simulink model "Copy_of_MPC_control"  (R2018a)
settings: Solver=FixedStepAuto  StartTime=0  StopTime=Tend  FixedStep=0.001  RelTol=5e-3
model workspace (MAT data in the model file):
  A_mu = 10
  B_reff = 8.386
  Cz = 7766.25
  DCT_Param : struct (value not decoded)
  D_reff = 0.25826
  Downshift_Speeds = [9.5625 12.9375 16.3125 19.6875 23.0625 26.4375 29.8125 33.1875 36.5625 39.9375 43.3125 46.6875 ... (28 elements, 4x7)]
  Pedal_Positions = [0.1 0.4 0.5 0.9]
  SUS : struct (value not decoded)
  Upshift_Speeds = [12.9375 16.3125 19.6875 33 26.4375 29.8125 33.1875 52.5 39.9375 43.3125 46.6875 77.25 ... (28 elements, 4x7)]
  VEH : struct (value not decoded)
  V_o = 16.7
  V_xlow = 1
  WH : struct (value not decoded)
  a = 1.4
  alpha_max = 1.5
  alpha_min = -1.5
  b = 1.8
  c_zo = 209651
  epsilon = 0.1
  h = 0.134
  path : struct (value not decoded)
  pio = 220000
  q_Fcx = 0
  q_Fz2 = 15.4
  q_Fzy = 0
  q_reo = 0.9974
  q_sx1 = -0.007764
  q_sx10 = 0.2824
  q_sx11 = 5.349
  q_sx12 = 0
  q_sx13 = 0
  q_sx14 = 0
  q_sx2 = 1.1915
  q_sx3 = 0.013948
  q_sx4 = 4.912
  q_sx5 = 1.02
  q_sx6 = 22.83
  q_sx7 = 0.7104
  q_sx8 = -0.023393
  q_sx9 = 0.6581
  q_sy1 = 0.00702
  q_sy2 = 0
  q_sy3 = 0.001515
  q_sy4 = 8.514e-05
  q_sy5 = 0
  q_sy6 = 0
  q_sy7 = 0.9008
  q_sy8 = -0.4089
  q_v1 = 0.0007742
  q_v2 = 0.04667
  r_Bx1 = 12.531
  r_Bx2 = 9.532
  r_Bx3 = 0
  r_By1 = 10.615
  r_By2 = 7.705
  r_By3 = 3.433e-06
  r_By4 = 0
  r_Cx1 = 1.019
  r_Cy1 = 1.0585
  r_Ex1 = -0.4487
  r_Ex2 = -0.4726
  r_Ey1 = 0.3132
  r_Ey2 = 7.63e-06
  r_Hx1 = 0.0002374
  r_Hy1 = 0.011646
  r_Hy2 = 7.63e-06
  r_Vy1 = 0.05654
  r_Vy2 = 7.63e-06
  r_Vy3 = 0
  r_Vy4 = 99.9
  r_Vy5 = 2
  r_Vy6 = 15.814
  r_o = 0.3135
  vehWidth = 2
  w = 1
symbols that are objects in the model workspace (value not decoded): VEH
undefined symbols (not defined in the file): C_Brake, C_Final, C_Front, C_Front_1, C_Front_2, C_Middle, C_out_Brake, C_out_Final, C_out_Front, C_out_Front_1, C_out_Front_2, C_out_Middle, Co, Cok_Brake, Cok_Final, Cok_Front_1, Cok_Front_2, Cok_Middle, Cso, D_out_Brake, D_out_Final, D_out_Front, D_out_Front_1, D_out_Front_2, D_out_Middle, Earlytochange, Earlytochange2, F, F_Brake, F_Final, F_Front, F_Front_1, F_Front_2, F_Middle, Fs, G_Brake, G_Final, G_Front_1, G_Front_2, G_Middle, G_sys_Brake, G_sys_Final, G_sys_Front, G_sys_Front_1, G_sys_Front_2, G_sys_Middle, Gd, Gd_Brake, Gd_Final, Gd_Front, Gd_Front_1, Gd_Front_2, Gd_Middle, Go, Gsd, Gso, H_Brake, H_Final, H_Front_1, H_Front_2 ... (+60)
libraries: simulink x10, sim3dlib x4, autolibutils x2, vehdynlibviscommon x2
(part 2 of 8)

== system Copy_of_MPC_control/Controllers/Brake Controller ==
  BrkPrsCmd : Inport
  xdot : Inport  Port=2
  kappa : Inport  Port=3
  Abs : Abs  ZeroCross=off
  Brake Pressure Control : Subsystem  Variant=on  OverrideUsingVariant=0
  Constant1 : Constant  Value=-20
  Gain3 : Gain
  Integrator2 : Integrator  LimitOutput=on  UpperSaturationLimit=1  LowerSaturationLimit=0
  Saturation : Saturate  UpperLimit=1  LowerLimit=0  ZeroCross=off
  Switch1 : Switch  Criteria=u2 > Threshold  Threshold=.1
  Vector Concatenate2 : Concatenate  NumInputs=4
  PCmd : Outport
  wires:
  Constant1/1 -> Switch1/3
  Gain3/1 -> Switch1/1
  Saturation/1 -> Brake Pressure Control/3(<Kappa>)  "Kappa"
  Brake Pressure Control/1(PCmd) -> PCmd/1
  kappa/1 -> Abs/1
  Integrator2/1 -> Vector Concatenate2/4, Vector Concatenate2/3, Vector Concatenate2/2, Vector Concatenate2/1
  xdot/1 -> Brake Pressure Control/2(xdot)
  Abs/1 -> Saturation/1
  Vector Concatenate2/1 -> Brake Pressure Control/1(Pref)  "Reference P"
  BrkPrsCmd/1 -> Switch1/2, Gain3/1
  Switch1/1 -> Integrator2/1

== system Copy_of_MPC_control/Controllers/ECU ==
  <Accel> : Inport
  Acc to Torque Request : Gain  Gain=150
  MATLAB Function : MATLAB Function  TreatAsAtomicUnit=on
  Stop Simulation : Stop
  Trq Cmd : Outport
  wires:
  Acc to Torque Request/1 -> Trq Cmd/1
  <Accel>/1 -> MATLAB Function/1("input ")
  MATLAB Function/2(output) -> Stop Simulation/1
  MATLAB Function/1(input) -> Acc to Torque Request/1

== system Copy_of_MPC_control/Controllers/Transmission Controller ==
  Acc : Inport
  EngSpd : Inport  Port=2  Unit=rad/s
  PropShaftSpd : Inport  Port=3
  10ms Function-Call Generator : simulink/Ports & Subsystems/Function-Call Generator  sample_time=Fcncal_transctrl_Ts  numberOfIterations=1
  Rate Transition{,1..3} (4 alike) : RateTransition
  Signal Specification : SignalSpecification  Unit=rpm
  TCM : Subsystem
  Unit Conversion : UnitConversion
  Gear : Outport
  wires:
  TCM/1(Gear Select) -> Rate Transition3/1
  Rate Transition/1 -> TCM/1(AccCmd)
  10ms Function-Call Generator/1 -> TCM/Trigger
  Acc/1 -> Rate Transition/1
  PropShaftSpd/1 -> Rate Transition2/1
  Rate Transition1/1 -> TCM/2(EngSpd)
  Rate Transition2/1 -> TCM/3(VehSpdFdbk)
  Rate Transition3/1 -> Gear/1
  Unit Conversion/1 -> Signal Specification/1
  Signal Specification/1 -> Rate Transition1/1  "EngSpd"
  EngSpd/1 -> Unit Conversion/1

== system Copy_of_MPC_control/Passenger Vehicle/Body, Suspension, Wheels ==
  note: 1) Add Subsystem or Model blocks as valid variant choices.
      | 2) You cannot connect blocks at this level. At simulation, connectivity is automatically
      | determined, based on the active variant and port name matching.
  WindXYZ : Inport
  Ground : Inport  Port=2  PortDimensions=4
  Friction : Inport  Port=3  PortDimensions=4
  WheelAngle : Inport  Port=4
  AxleTrq : Inport  Port=5
  BrkPrs : Inport  Port=6
  PassVeh14DOF : ModelReference  DisableCoverage=on  ModelNameDialog=PassVeh14DOF  VariantControl=3  ModelReferenceVersion=1.200
  PassVeh7DOF : ModelReference  DisableCoverage=on  ModelNameDialog=PassVeh7DOF  VariantControl=1  ModelReferenceVersion=1.152
  xdot : Outport
  ydot : Outport  Port=2
  X : Outport  Port=3
  Y : Outport  Port=4
  Z : Outport  Port=5
  Xdot : Outport  Port=6
  Ydot : Outport  Port=7
  phi : Outport  Port=8
  theta : Outport  Port=9
  psi : Outport  Port=10
  p : Outport  Port=11
  q : Outport  Port=12
  r : Outport  Port=13
  ay : Outport  Port=14
  kappa : Outport  Port=15
  zAxle : Outport  Port=16
  omega : Outport  Port=17
  ZHP : Outport  Port=18  Unit=m
  XWheel : Outport  Port=19
  YWheel : Outport  Port=20

== system Copy_of_MPC_control/Passenger Vehicle/Engine ==
  note: 1) Add Subsystem or Model blocks as valid variant choices.
      | 2) You cannot connect blocks at this level. At simulation, connectivity is automatically
      | determined, based on the active variant and port name matching.
  TrqCmd : Inport
  EngSpd : Inport  Port=2  Unit=rad/s
  Ideal Mapped Engine : ModelReference  DisableCoverage=on  ModelNameDialog=SiMappedEngineV  VariantControl=0  ModelReferenceVersion=1.335
  EngTrq : Outport

== system Copy_of_MPC_control/Passenger Vehicle/Steering, Transmission, Driveline and Brakes ==
  note: 1) Add Subsystem or Model blocks as valid variant choices.
      | 2) You cannot connect blocks at this level. At simulation, connectivity is automatically
      | determined, based on the active variant and port name matching.
  SteerHWCmd : Inport
  EngTrq : Inport  Port=2
  GearCmd : Inport  Port=3  OutDataTypeStr=int8
  BrkPrsCmd : Inport  Port=4  PortDimensions=4
  omega : Inport  Port=5
  Driveline Ideal Fixed Gear : ModelReference  DisableCoverage=on  ModelNameDialog=Driveline  VariantControl=0  ModelReferenceVersion=1.207
  WhlAng : Outport
  AxlTrq : Outport  Port=2
  BrkPrs : Outport  Port=3  PortDimensions=4
  EngSpd : Outport  Port=4  Unit=rad/s
  PropShftSpd : Outport  Port=5

== system Copy_of_MPC_control/Passenger Vehicle/Subsystem ==
  Env : Inport
  Driveline : Inport  Port=2
  Bus Selector1 : BusSelector  OutputSignals=Gnd.z.G_FL_z,Gnd.z.G_FR_z,Gnd.z.G_RL_z,Gnd.z.G_RR_z
  Bus Selector2 : BusSelector  OutputSignals=Wind
  Bus Selector3 : BusSelector  OutputSignals=Gnd.mu.mu_FL,Gnd.mu.mu_FR,Gnd.mu.mu_RL,Gnd.mu.mu_RR
  Bus Selector4 : BusSelector  OutputSignals=WhlAng,AxlTrq,BrkPrs
  Vector Concatenate : Concatenate  NumInputs=4
  Vector Concatenate1 : Concatenate  NumInputs=4
  Wind : Outport
  Gnd : Outport  Port=2
  mu : Outport  Port=3
  WhlAng : Outport  Port=4
  AxleTrq : Outport  Port=5
  BrkPrs : Outport  Port=6
  wires:
  Env/1 -> Bus Selector3/1, Bus Selector1/1, Bus Selector2/1
  Bus Selector2/1 -> Wind/1  "<Wind>"
  Bus Selector3/1 -> Vector Concatenate/1  "<mu_FL>"
  Bus Selector3/2 -> Vector Concatenate/2  "<mu_FR>"
  Bus Selector3/3 -> Vector Concatenate/3  "<mu_RL>"
  Bus Selector3/4 -> Vector Concatenate/4  "<mu_RR>"
  Vector Concatenate/1 -> mu/1
  Bus Selector1/1 -> Vector Concatenate1/1  "<G_FL_z>"
  Bus Selector1/2 -> Vector Concatenate1/2  "<G_FR_z>"
  Bus Selector1/3 -> Vector Concatenate1/3  "<G_RL_z>"
  Bus Selector1/4 -> Vector Concatenate1/4  "<G_RR_z>"
  Vector Concatenate1/1 -> Gnd/1
  Driveline/1 -> Bus Selector4/1
  Bus Selector4/2 -> AxleTrq/1  "<AxlTrq>"
  Bus Selector4/1 -> WhlAng/1  "<WhlAng>"
  Bus Selector4/3 -> BrkPrs/1  "<BrkPrs>"

== system Copy_of_MPC_control/Passenger Vehicle/Subsystem1 ==
  WhlAng : Inport
  AxlTrq : Inport  Port=2
  BrkPrs : Inport  Port=3
  EngSpd : Inport  Port=4
  PropShftSpd : Inport  Port=5
  Bus Creator1 : BusCreator  Inputs=5
  Driveline : Outport
  wires:
  Bus Creator1/1 -> Driveline/1  "Driveline"
  PropShftSpd/1 -> Bus Creator1/5  "PropShftSpd"
  AxlTrq/1 -> Bus Creator1/2  "AxlTrq"
  WhlAng/1 -> Bus Creator1/1  "WhlAng"
  EngSpd/1 -> Bus Creator1/4  "EngSpd"
  BrkPrs/1 -> Bus Creator1/3  "BrkPrs"

== system Copy_of_MPC_control/Passenger Vehicle/Subsystem2 ==
  Cntrl : Inport
  SteerCmd : Inport  Port=2
  EngTrqCmd : Inport  Port=3
  Wheels : Inport  Port=4
  Bus Selector1 : BusSelector  OutputSignals=Steer
  Bus Selector2 : BusSelector  OutputSignals=omega
  Bus Selector3 : BusSelector  OutputSignals=Transmission.GearCmd,Brake.PrsCmd
  Bus Selector4 : BusSelector  OutputSignals=EngTrq
  Steer : Outport
  EngTrq : Outport  Port=2
  GearCmd : Outport  Port=3
  PrsCmd : Outport  Port=4
  omega : Outport  Port=5
  wires:
  Cntrl/1 -> Bus Selector3/1
  Bus Selector3/1 -> GearCmd/1  "<GearCmd>"
  SteerCmd/1 -> Bus Selector1/1
  Wheels/1 -> Bus Selector2/1
  Bus Selector2/1 -> omega/1  "<omega>"
  Bus Selector3/2 -> PrsCmd/1  "<PrsCmd>"
  EngTrqCmd/1 -> Bus Selector4/1
  Bus Selector1/1 -> Steer/1  "<Steer>"
  Bus Selector4/1 -> EngTrq/1  "<EngTrq>"

== system Copy_of_MPC_control/Passenger Vehicle/Subsystem3 ==
  Cntrl : Inport
  Driveline : Inport  Port=2
  Bus Selector : BusSelector  OutputSignals=ECU.EngTrqCmd
  Bus Selector1 : BusSelector  OutputSignals=EngSpd
  EngTrqCmd : Outport
  EngSpd : Outport  Port=2
  wires:
  Driveline/1 -> Bus Selector1/1
  Cntrl/1 -> Bus Selector/1
  Bus Selector/1 -> EngTrqCmd/1  "<EngTrqCmd>"
  Bus Selector1/1 -> EngSpd/1  "<EngSpd>"

== system Copy_of_MPC_control/Passenger Vehicle/Subsystem4 ==
  xdot : Inport
  ydot : Inport  Port=2
  X : Inport  Port=3
  Y : Inport  Port=4
  Z : Inport  Port=5
  Xdot : Inport  Port=6
  Ydot : Inport  Port=7
  phi : Inport  Port=8
  theta : Inport  Port=9
  psi : Inport  Port=10
  p : Inport  Port=11
  q : Inport  Port=12
  r : Inport  Port=13
  ay : Inport  Port=14
  kappa : Inport  Port=15
  zAxle : Inport  Port=16
  omega : Inport  Port=17
  ZHP : Inport  Port=18
  XWheel : Inport  Port=19
  YWheel : Inport  Port=20
  Bus Creator : BusCreator  Inputs=15
  Bus Creator3 : BusCreator  Inputs=5
  Chassis : Outport
  Wheels : Outport  Port=2
  wires:
  X/1 -> Bus Creator/3  "X"
  psi/1 -> Bus Creator/10  "psi"
  ydot/1 -> Bus Creator/2  "ydot"
  Z/1 -> Bus Creator/5  "Z"
  Bus Creator/1 -> Chassis/1  "Chassis"
  Y/1 -> Bus Creator/4  "Y"
  xdot/1 -> Bus Creator/1  "xdot"
  r/1 -> Bus Creator/13  "r"
  ay/1 -> Bus Creator/14  "ay"
  omega/1 -> Bus Creator3/3  "omega"
  zAxle/1 -> Bus Creator3/2  "zAxle"
  kappa/1 -> Bus Creator3/1  "kappa"
  Bus Creator3/1 -> Wheels/1  "Wheels"
  theta/1 -> Bus Creator/9  "theta"
  phi/1 -> Bus Creator/8  "phi"
  Xdot/1 -> Bus Creator/6  "Xdot"
  Ydot/1 -> Bus Creator/7  "Ydot"
  ZHP/1 -> Bus Creator/15  "ZHP"
  p/1 -> Bus Creator/11  "p"
  q/1 -> Bus Creator/12  "q"
  YWheel/1 -> Bus Creator3/5  "YWheel"
  XWheel/1 -> Bus Creator3/4  "XWheel"

== system Copy_of_MPC_control/Passenger Vehicle/Subsystem5 ==
  "EngTrq " : Inport
  Bus Creator : BusCreator  Inputs=1
  Eng : Outport
  wires:
  "EngTrq "/1 -> Bus Creator/1  "EngTrq"
  Bus Creator/1 -> Eng/1

== system Copy_of_MPC_control/Visualization/3D Engine ==
  note: 1) Add Subsystem or Model blocks as valid variant choices.
      | 2) You cannot connect blocks at this level. At simulation, connectivity is automatically
      | determined, based on the active variant and port name matching.
  VehFdbk : Inport
  3D Engine : Subsystem  VariantControl=1
  3D Engine Disabled : Subsystem  VariantControl=0

== system Copy_of_MPC_control/Visualization/Acceleration Cmd ==

== system Copy_of_MPC_control/Visualization/Brake Cmd ==

== system Copy_of_MPC_control/Visualization/Engine Tach [rpm] ==

== system Copy_of_MPC_control/Visualization/Handwheel Angle [deg] ==

== system Copy_of_MPC_control/Visualization/Lateral Acceleration [g] ==

== system Copy_of_MPC_control/Visualization/Speed [mph] ==

== system Copy_of_MPC_control/Visualization/Vehicle XY Plotter ==
  VehFdbk : Inport
  Bus Selector1 : BusSelector  OutputSignals=Body.phi,Body.theta,Body.psi  OutputAsBus=on
  Bus Selector2 : BusSelector  OutputSignals=Driveline.WhlAng  OutputAsBus=on
  Bus Selector3 : BusSelector  OutputSignals=Body.X,Body.Y,Body.Z  OutputAsBus=on
  Bus Selector4 : BusSelector  OutputSignals=Body.Xdot,Body.Ydot  OutputAsBus=on
  Bus to Vector{,1..3} (4 alike) : BusToVector
  Ground : Ground
  Rate Transition{1..2,5..6} (4 alike) : RateTransition  OutPortSampleTime=pltDT
  Vector Concatenate : Concatenate
  Vehicle XY Plotter : vehdynlibviscommon/Vehicle XY Plotter  bufferSize=bufferSize  w=w  a=a  b=b
  wires:
  Bus to Vector2/1 -> Rate Transition1/1  "InertCGDisp"
  Rate Transition5/1 -> Vehicle XY Plotter/1
  Bus Selector4/1 -> Bus to Vector1/1
  Rate Transition1/1 -> Vehicle XY Plotter/2
  Rate Transition6/1 -> Vehicle XY Plotter/3
  Vector Concatenate/1 -> Rate Transition6/1  "InertCGVel"
  Bus Selector1/1 -> Bus to Vector2/1
  Bus to Vector/1 -> Rate Transition5/1  "InertCGDisp"
  Bus Selector3/1 -> Bus to Vector/1
  Bus to Vector1/1 -> Vector Concatenate/1
  Ground/1 -> Vector Concatenate/2
  Bus to Vector3/1 -> Rate Transition2/1
  Bus Selector2/1 -> Bus to Vector3/1
  VehFdbk/1 -> Bus Selector1/1, Bus Selector2/1, Bus Selector4/1, Bus Selector3/1
  Rate Transition2/1 -> Vehicle XY Plotter/4

== system Copy_of_MPC_control/all_system/Controllers1 ==
  Pedals : Inport
  VehFdbk : Inport  Port=2
  Brake Controller : Subsystem
  Bus Creator : BusCreator  Inputs=1
  Bus Creator1 : BusCreator  Inputs=1
  Bus Creator2 : BusCreator  Inputs=1
  Bus Creator3 : BusCreator  Inputs=3
  Bus Selector : BusSelector  OutputSignals=Body.xdot,Wheels.kappa
  Bus Selector1 : BusSelector  OutputSignals=Driveline.EngSpd,Driveline.PropShftSpd
  Bus Selector2 : BusSelector  OutputSignals=Accel,Brake
  ECU : Subsystem
  Transmission Controller : Subsystem
  Controller : Outport
  wires:
  Transmission Controller/1(Gear) -> Bus Creator1/1  "GearCmd"
  Bus Selector/2 -> Brake Controller/3(kappa)  "<kappa>"
  ECU/1(Trq Cmd) -> Bus Creator/1  "EngTrqCmd"
  Brake Controller/1(PCmd) -> Bus Creator2/1  "PrsCmd"
  VehFdbk/1 -> Bus Selector/1, Bus Selector1/1
  Bus Selector/1 -> Brake Controller/2(xdot)  "<xdot>"
  Bus Selector1/1 -> Transmission Controller/2(EngSpd)  "<EngSpd>"
  Bus Selector1/2 -> Transmission Controller/3(PropShaftSpd)  "<PropShftSpd>"
  Pedals/1 -> Bus Selector2/1
  Bus Selector2/1 -> Transmission Controller/1(Acc), ECU/1(<Accel>)  "<Accel>"
  Bus Selector2/2 -> Brake Controller/1(BrkPrsCmd)  "<Brake>"
  Bus Creator/1 -> Bus Creator3/1  "ECU"
  Bus Creator1/1 -> Bus Creator3/2  "Transmission"
  Bus Creator2/1 -> Bus Creator3/3  "Brake"
  Bus Creator3/1 -> Controller/1  "Controller"

== system Copy_of_MPC_control/all_system/Dataselect1 ==
  Clock15 : Clock
  Constant3 : Constant  Value=Statechange
  Constant4 : Constant  Value=Statechange2
  Dataselect : MATLAB Function  TreatAsAtomicUnit=on
  DS : Outport
  wires:
  Constant4/1 -> Dataselect/3(Statechange2)
  Clock15/1 -> Dataselect/1(timing)
  Constant3/1 -> Dataselect/2(Statechange)
  Dataselect/1(select) -> DS/1

== system Copy_of_MPC_control/all_system/Environment1 ==
  Bus Creator : BusCreator  Inputs=4
  Bus Creator1 : BusCreator  Inputs=2
  Bus Creator2 : BusCreator  Inputs=4
  Bus Creator3 : BusCreator  Inputs=2
  Constant1 : Constant  Value=zeros(4,1)
  Constant3 : Constant  Value=0
  Constant4 : Constant  Value=0
  Constant5 : Constant  Value=0
  Demux : Demux
  Demux1 : Demux
  Friction : Constant  Value=ones(4,1).*1
  Vector Concatenate : Concatenate  NumInputs=3
  Env : Outport
  wires:
  Constant1/1 -> Demux/1
  Bus Creator2/1 -> Bus Creator3/2  "mu"
  Bus Creator/1 -> Bus Creator3/1  "z"
  Demux/2 -> Bus Creator/2  "G_FR_z"
  Demux/3 -> Bus Creator/3  "G_RL_z"
  Constant5/1 -> Vector Concatenate/3  "Z"
  Demux/1 -> Bus Creator/1  "G_FL_z"
  Vector Concatenate/1 -> Bus Creator1/1  "Wind"
  Constant3/1 -> Vector Concatenate/1  "X"
  Demux/4 -> Bus Creator/4  "G_RR_z"
  Constant4/1 -> Vector Concatenate/2  "Y"
  Demux1/3 -> Bus Creator2/3  "mu_RL"
  Demux1/4 -> Bus Creator2/4  "mu_RR"
  Demux1/2 -> Bus Creator2/2  "mu_FR"
  Demux1/1 -> Bus Creator2/1  "mu_FL"
  Friction/1 -> Demux1/1
  Bus Creator3/1 -> Bus Creator1/2  "Gnd"
  Bus Creator1/1 -> Env/1

== system Copy_of_MPC_control/all_system/Final Observer2 ==
  Final_switch : Inport
  U : Inport  Port=2
  Y : Inport  Port=3
  Rs : Inport  Port=4
  U_delay : Inport  Port=5
  r(k-1) : Inport  Port=6
  r(k) : Inport  Port=7
  Initial position : Inport  Port=8
  Initial Velocities : Inport  Port=9
  Initial HeadingAngles : Inport  Port=10
  Tsim : Inport  Port=11
  LastTsim : Inport  Port=12
  Enable : EnablePort
  C_Final2 : Gain  Gain=C_Final  Multiplication=Matrix(K*u) (u vector)
  Clock : Clock
  Clock1 : Clock
  Delay : Delay  DelayLength=1  InitialConditionSource=Input port  InitialCondition=0  ExternalReset=Falling  SampleTime=Ts
      settings: InputPortMap=u0,r5,p4
  Delay1 : Delay  DelayLength=1  InitialConditionSource=Input port  InitialCondition=0  ExternalReset=Falling  SampleTime=Ts
      settings: InputPortMap=u0,r5,p4
  Final_switch3 : InportShadow
  Final_switch4 : InportShadow
  Gd_Final : Gain  Gain=Gd_Final  Multiplication=Matrix(K*u) (u vector)
  Hd_Final : Gain  Gain=Hd_Final  Multiplication=Matrix(K*u) (u vector)
  Ld_Final1 : Gain  Gain=Ld_Final  Multiplication=Matrix(K*u) (u vector)
  Ld_Final2 : Gain  Gain=Ld_Final  Multiplication=Matrix(K*u) (u vector)
  Subsystem : Subsystem
  Sum4 : Sum  Inputs=+++
  Switch : Switch  Threshold=Timetochange2
  Switch1 : Switch  Threshold=Timetochange2
  To Workspace : ToWorkspace  VariableName=FW  SaveFormat=Timeseries  SampleTime=Ts
  yhat : Outport
  xhat_delay : Outport  Port=2
  u_delay : Outport  Port=3
  xhat : Outport  Port=4
  wires:
  Switch/1 -> Delay1/1
  U/1 -> Switch/1
  Gd_Final/1 -> Sum4/3
  Delay/1 -> Gd_Final/1, xhat_delay/1
  Ld_Final1/1 -> Sum4/1
  Hd_Final/1 -> Sum4/2
  C_Final2/1 -> yhat/1
  Delay1/1 -> u_delay/1, Hd_Final/1
  Sum4/1 -> Subsystem/11(Xh_sim), xhat/1, C_Final2/1, Delay/1
  Y/1 -> Switch1/1
  Switch1/1 -> Ld_Final1/1
  r(k-1)/1 -> Ld_Final2/1, Subsystem/9(r(k-1))
  Ld_Final2/1 -> Delay/3
  r(k)/1 -> Subsystem/10(r(k))
  Rs/1 -> Subsystem/2(Rs)
  U_delay/1 -> Delay1/3, Subsystem/3(U_delay)
  Initial position/1 -> Subsystem/4(Initial position)
  Initial Velocities/1 -> Subsystem/5(Initial Velocities)
  Initial HeadingAngles/1 -> Subsystem/6(Initial HeadingAngles)
  Tsim/1 -> Subsystem/7(Tsim)
  LastTsim/1 -> Subsystem/8(LastTsim)
  Subsystem/1(Y) -> Switch1/3
  Subsystem/2(U) -> Switch/3
  Final_switch/1 -> To Workspace/1, Subsystem/1(Initial trigger)
  Final_switch3/1 -> Delay1/2
  Final_switch4/1 -> Delay/2
  Clock/1 -> Switch/2
  Clock1/1 -> Switch1/2

== system Copy_of_MPC_control/all_system/Final_simulator1 ==
  Rs_V : Inport
  Rs : Inport  Port=2
  r(k)Middle : Inport  Port=3
  r(k-1)Middle : Inport  Port=4
  udelayMiddle : Inport  Port=5
  PositionfromMiddle : Inport  Port=6
  VelocitiesfromMiddle : Inport  Port=7
  HeadingAnglesfromMiddle : Inport  Port=8
  T_sim : Inport  Port=9
  LastT_sim : Inport  Port=10
  Enable : EnablePort
  Mpc_Simulator_Final : Subsystem
  Simulator_Final : Subsystem
  VH2P : Subsystem
  YV_update_Np : Subsystem  TreatAsAtomicUnit=on
  Velocity : Outport
  Heading_angle : Outport  Port=2
  U : Outport  Port=3
  PositionfromFinal : Outport  Port=4
  Rs_heading_angle : Outport  Port=5
  Vup : Outport  Port=6
  SyetemError : Outport  Port=7
  Ldterm : Outport  Port=8
  OutputError : Outport  Port=9
  yhat : Outport  Port=10
  lambda : Outport  Port=11
  wires:
  VH2P/1(Position) -> YV_update_Np/1(XY_sim), PositionfromFinal/1
  Simulator_Final/1(velocity_sim) -> YV_update_Np/2(Velocity_sim), Velocity/1, VH2P/1(Velocities)
  Simulator_Final/2(yaw_sim) -> YV_update_Np/3(Heading_sim), VH2P/2(HeadingAngles), Heading_angle/1
  YV_update_Np/2(Heading angle) -> Rs_heading_angle/1, Mpc_Simulator_Final/2(Yup)
  Mpc_Simulator_Final/1(U) -> Simulator_Final/1(u_simulator), U/1
  Simulator_Final/7(xh_simulator) -> Mpc_Simulator_Final/5(Xh_sim)
  Mpc_Simulator_Final/2(Ref) -> Simulator_Final/2(Ref)
  Rs_V/1 -> Mpc_Simulator_Final/3(Rs_V)
  Simulator_Final/5(OutputError) -> OutputError/1
  Simulator_Final/4(Ldterm) -> Ldterm/1
  Simulator_Final/3(SystemError) -> SyetemError/1
  Simulator_Final/6(yhat) -> yhat/1
  YV_update_Np/1(Velocity) -> Mpc_Simulator_Final/1(Vup), Vup/1
  PositionfromMiddle/1 -> VH2P/3(PositionfromMiddle)
  r(k-1)Middle/1 -> Simulator_Final/4(r(k-1)Middle)
  r(k)Middle/1 -> Simulator_Final/3(r(k)Middle)
  udelayMiddle/1 -> Simulator_Final/5(udelayMiddle)
  VelocitiesfromMiddle/1 -> VH2P/4(VelocitiesfromMiddle)
  HeadingAnglesfromMiddle/1 -> VH2P/5(HeadingAnglesfromMiddle)
  T_sim/1 -> VH2P/6(T_sim)
  Rs/1 -> Mpc_Simulator_Final/4(Rs)
  LastT_sim/1 -> VH2P/7(LastT_sim)
  Mpc_Simulator_Final/3(lambda) -> lambda/1

== system Copy_of_MPC_control/all_system/Final_simulator_ operating_time1 ==
  Clock14 : Clock
  Constant1 : Constant  Value=Earlytochange2
  MATLAB Function2 : MATLAB Function  TreatAsAtomicUnit=on
  state : Outport
  wires:
  Constant1/1 -> MATLAB Function2/2(Earlytochange2)
  MATLAB Function2/1(state) -> state/1
  Clock14/1 -> MATLAB Function2/1(timing)

== system Copy_of_MPC_control/all_system/Front Observer2 ==
  Y : Inport
  U : Inport  Port=2
  Enable : EnablePort
  Cso : Gain  Gain=Cso  Multiplication=Matrix(K*u) (u vector)
  "Gsd " : Gain  Gain=Gsd  Multiplication=Matrix(K*u) (u vector)
  Hsd : Gain  Gain=Hsd  Multiplication=Matrix(K*u) (u vector)
  Lsd : Gain  Gain=Lsd  Multiplication=Matrix(K*u) (u vector)
  Sum3 : Sum  Inputs=+++
  Unit Delay2 : UnitDelay  InitialCondition=xho  SampleTime=Ts
  Unit Delay3 : UnitDelay  InitialCondition=[0;0]  SampleTime=Ts
  yhat : Outport
  xhat_delay : Outport  Port=2
  u_delay : Outport  Port=3
  xhat : Outport  Port=4
  wires:
  Unit Delay3/1 -> u_delay/1, Hsd/1
  "Gsd "/1 -> Sum3/3
  Lsd/1 -> Sum3/1
  Unit Delay2/1 -> xhat_delay/1, "Gsd "/1
  U/1 -> Unit Delay3/1
  Hsd/1 -> Sum3/2
  Y/1 -> Lsd/1
  Cso/1 -> yhat/1
  Sum3/1 -> xhat/1, Cso/1, Unit Delay2/1

== system Copy_of_MPC_control/all_system/Front_simulator1 ==
  Rs_V : Inport
  Enable : EnablePort
  From Workspace : FromWorkspace  VariableName=Rs  SampleTime=Ts
  Mpc_Simulator_Front : Subsystem
  Simulator_Front : Subsystem
  VH2P : Subsystem
  YV_update_Np : Subsystem  TreatAsAtomicUnit=on
  Velocity : Outport
  Heading_angle : Outport  Port=2
  U : Outport  Port=3
  Position : Outport  Port=4
  Rs_heading_angle : Outport  Port=5
  Vup : Outport  Port=6
  SyetemError : Outport  Port=7
  Ldterm : Outport  Port=8
  OutputError : Outport  Port=9
  yhat : Outport  Port=10
  r(k+1)Front : Outport  Port=11
  lambda : Outport  Port=12
  wires:
  VH2P/1(Position) -> YV_update_Np/1(XY_sim), Position/1
  Simulator_Front/1(velocity_sim) -> YV_update_Np/2(Velocity_sim), Velocity/1, VH2P/1(Velocities)
  Simulator_Front/2(yaw_sim) -> YV_update_Np/3(Heading_sim), VH2P/2(HeadingAngles), Heading_angle/1
  YV_update_Np/2(Heading angle) -> Mpc_Simulator_Front/2(Yup), Rs_heading_angle/1
  Mpc_Simulator_Front/1(U) -> U/1, Simulator_Front/1(u_simulator)
  Simulator_Front/3(xh_simulator) -> Mpc_Simulator_Front/4(Xh_sim)
  Mpc_Simulator_Front/2(Ref) -> r(k+1)Front/1, Simulator_Front/2(Ref)
  Rs_V/1 -> Mpc_Simulator_Front/3(Rs_V)
  Simulator_Front/6(OutputError) -> OutputError/1
  Simulator_Front/5(Ldterm) -> Ldterm/1
  Simulator_Front/4(SystemError) -> SyetemError/1
  Simulator_Front/7(yhat) -> yhat/1
  YV_update_Np/1(Velocity) -> Mpc_Simulator_Front/1(Vup), Vup/1
  From Workspace/1 -> Mpc_Simulator_Front/5(Rs)
  Mpc_Simulator_Front/3(lambda) -> lambda/1

== system Copy_of_MPC_control/all_system/Front_simulator_ operating_time1 ==
  Clock9 : Clock
  Constant : Constant  Value=Statechange
  MATLAB Function1 : MATLAB Function  TreatAsAtomicUnit=on
  state : Outport
  wires:
  MATLAB Function1/1(state) -> state/1
  Clock9/1 -> MATLAB Function1/1(timing)
  Constant/1 -> MATLAB Function1/2(Statechange)

== system Copy_of_MPC_control/all_system/Longitudinal Driver1 ==
  In1 : Inport  SampleTime=Tf
  In2 : Inport  Port=2  SampleTime=Tf
  In3 : Inport  Port=3  SampleTime=Tf
  Bus Creator1 : BusCreator  Inputs=3
  To Workspace : ToWorkspace  VariableName=Brake  SampleTime=Tf
  To Workspace1 : ToWorkspace  VariableName=Steer  SampleTime=-1
  To Workspace2 : ToWorkspace  VariableName=Acceleration  SampleTime=Tf
  Driver : Outport
  wires:
  Bus Creator1/1 -> Driver/1
  In2/1 -> To Workspace2/1, Bus Creator1/2  "Accel"
  In3/1 -> Bus Creator1/3, To Workspace/1  "Brake"
  In1/1 -> To Workspace1/1, Bus Creator1/1  "Steer"

== system Copy_of_MPC_control/all_system/Middle Observer2 ==
  U : Inport
  Y : Inport  Port=2
  Rs : Inport  Port=3
  Initial position : Inport  Port=4
  U_delay : Inport  Port=5
  r(k-1) : Inport  Port=6
  r(k) : Inport  Port=7
  Initial Velocities : Inport  Port=8
  Initial HeadingAngles : Inport  Port=9
  Tsim : Inport  Port=10
  LastTsim : Inport  Port=11
  Enable : EnablePort
  Clock : Clock
  Clock1 : Clock
  Co : Gain  Gain=Co  Multiplication=Matrix(K*u) (u vector)
  Delay : Delay  DelayLength=1  InitialConditionSource=Input port  InitialCondition=0  SampleTime=Ts
      settings: InputPortMap=u0,p4
  Delay1 : Delay  DelayLength=1  InitialConditionSource=Input port  InitialCondition=0  SampleTime=Ts
      settings: InputPortMap=u0,p4
  Gd : Gain  Gain=Gd  Multiplication=Matrix(K*u) (u vector)
  Hd : Gain  Gain=Hd  Multiplication=Matrix(K*u) (u vector)
  Ld : Gain  Gain=Ld  Multiplication=Matrix(K*u) (u vector)
  Ld1 : Gain  Gain=Ld  Multiplication=Matrix(K*u) (u vector)
  Observer_state2 : Subsystem
  Subsystem : Subsystem
  Sum4 : Sum  Inputs=+++
  Switch : Switch  Threshold=Timetochange
  Switch1 : Switch  Threshold=Timetochange
  To Workspace1 : ToWorkspace  VariableName=observer_simulator_xhstate  SampleTime=Ts
  To Workspace2 : ToWorkspace  VariableName=observer_simulator_u  SampleTime=Ts
  yhat : Outport
  xhat_delay : Outport  Port=2
  u_delay : Outport  Port=3
  xhat : Outport  Port=4
  wires:
  Delay1/1 -> u_delay/1, To Workspace2/1, Hd/1
  Sum4/1 -> xhat/1, Subsystem/10(xhat), Co/1, Delay/1
  Co/1 -> yhat/1
  Hd/1 -> Sum4/2
  Gd/1 -> Sum4/3
  Ld/1 -> Sum4/1
  Delay/1 -> To Workspace1/1, Gd/1, xhat_delay/1
  U/1 -> Switch/1
  Switch/1 -> Delay1/1
  Ld1/1 -> Delay/2
  Y/1 -> Switch1/1
  Switch1/1 -> Ld/1
  Clock/1 -> Switch/2
  Clock1/1 -> Switch1/2
  Rs/1 -> Subsystem/1(Rs)
  Initial position/1 -> Subsystem/5(Initial position)
  Subsystem/2(U) -> Switch/3
  Observer_state2/1(state) -> Subsystem/Enable
  Subsystem/1(Y) -> Switch1/3
  r(k-1)/1 -> Ld1/1, Subsystem/4(r(k-1))
  U_delay/1 -> Delay1/2, Subsystem/2(U_delay)
  r(k)/1 -> Subsystem/3(r(k))
  Initial Velocities/1 -> Subsystem/6(Initial Velocities)
  Initial HeadingAngles/1 -> Subsystem/7(Initial HeadingAngles)
  Tsim/1 -> Subsystem/8(Tsim)
  LastTsim/1 -> Subsystem/9(LastTsim)

== system Copy_of_MPC_control/all_system/Middle_simulator1 ==
  Rs_V : Inport
  Rs : Inport  Port=2
  r(k)Front : Inport  Port=3
  r(k-1)Front : Inport  Port=4
  udelayFront : Inport  Port=5
  PositionfromFront : Inport  Port=6
  VelocitiesfromFront : Inport  Port=7
  HeadingAnglesfromFront : Inport  Port=8
  T_sim : Inport  Port=9
  LastT_sim : Inport  Port=10
  Enable : EnablePort
  Mpc_Simulator_Middle : Subsystem
  Simulator_Middle : Subsystem
  VH2P : Subsystem
  YV_update_Np : Subsystem  TreatAsAtomicUnit=on
  Velocity : Outport
  Heading_angle : Outport  Port=2
  U : Outport  Port=3
  PositionfromMiddle : Outport  Port=4
  Rs_heading_angle : Outport  Port=5
  Vup : Outport  Port=6
  SyetemError : Outport  Port=7
  Ldterm : Outport  Port=8
  OutputError : Outport  Port=9
  yhat : Outport  Port=10
  r(k+1)Middle : Outport  Port=11
  lambda : Outport  Port=12
  wires:
  VH2P/1(Position) -> YV_update_Np/1(XY_sim), PositionfromMiddle/1
  Simulator_Middle/1(velocity_sim) -> YV_update_Np/2(Velocity_sim), Velocity/1, VH2P/1(Velocities)
  Simulator_Middle/2(yaw_sim) -> YV_update_Np/3(Heading_sim), VH2P/2(HeadingAngles), Heading_angle/1
  YV_update_Np/2(Heading angle) -> Mpc_Simulator_Middle/2(Yup), Rs_heading_angle/1
  Mpc_Simulator_Middle/1(U) -> U/1, Simulator_Middle/1(u_simulator)
  Simulator_Middle/7(xh_simulator) -> Mpc_Simulator_Middle/5(Xh_sim)
  Rs_V/1 -> Mpc_Simulator_Middle/3(Rs_V)
  Simulator_Middle/5(OutputError) -> OutputError/1
  Simulator_Middle/4(Ldterm) -> Ldterm/1
  Simulator_Middle/3(SystemError) -> SyetemError/1
  Simulator_Middle/6(yhat) -> yhat/1
  YV_update_Np/1(Velocity) -> Mpc_Simulator_Middle/1(Vup), Vup/1
  r(k)Front/1 -> Simulator_Middle/3(r(k))
  r(k-1)Front/1 -> Simulator_Middle/4(r(k-1))
  Mpc_Simulator_Middle/2(Ref) -> r(k+1)Middle/1, Simulator_Middle/2(Ref)
  Rs/1 -> Mpc_Simulator_Middle/4(Rs)
  VelocitiesfromFront/1 -> VH2P/4(VelocitiesfromFront)
  HeadingAnglesfromFront/1 -> VH2P/5(HeadingAnglesfromFront)
  T_sim/1 -> VH2P/6(T_sim)
  PositionfromFront/1 -> VH2P/3(PositionfromFront)
  udelayFront/1 -> Simulator_Middle/5(udelayFront)
  LastT_sim/1 -> VH2P/7(LastT_sim)
  Mpc_Simulator_Middle/3(lambda) -> lambda/1

== system Copy_of_MPC_control/all_system/Middle_simulator_ operating_time1 ==
  Clock14 : Clock
  Constant1 : Constant  Value=Timetochange
  Constant2 : Constant  Value=Statechange2
  MATLAB Function2 : MATLAB Function  TreatAsAtomicUnit=on
  state : Outport
  wires:
  Constant1/1 -> MATLAB Function2/2(Timetochange)
  MATLAB Function2/1(state) -> state/1
  Clock14/1 -> MATLAB Function2/1(timing)
  Constant2/1 -> MATLAB Function2/3(Statechange2)

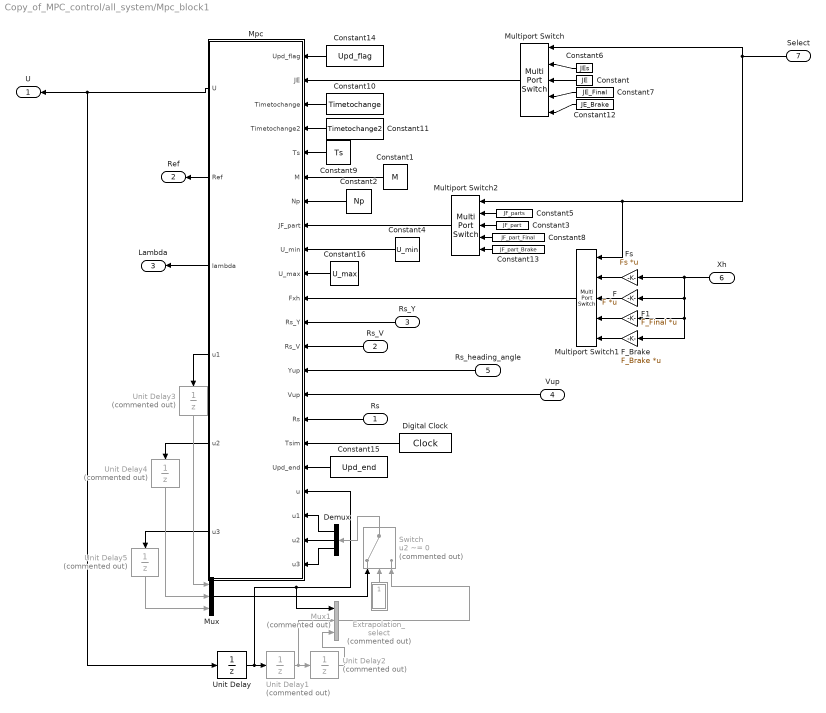
== system Copy_of_MPC_control/all_system/Mpc_block1 ==
  Rs : Inport  SampleTime=Ts  LockScale=on
  Rs_V : Inport  Port=2  SampleTime=Ts  LockScale=on
  Rs_Y : Inport  Port=3  SampleTime=Ts  LockScale=on
  Vup : Inport  Port=4  SampleTime=Ts
  Rs_heading_angle : Inport  Port=5  SampleTime=Ts  LockScale=on
  Xh : Inport  Port=6
  Select : Inport  Port=7
  Constant : Constant  Value=JE  VectorParams1D=off  SampleTime=-1
  Constant1 : Constant  Value=M  VectorParams1D=off  SampleTime=-1
  Constant10 : Constant  Value=Timetochange  VectorParams1D=off  SampleTime=-1
  Constant11 : Constant  Value=Timetochange2  VectorParams1D=off  SampleTime=-1
  Constant12 : Constant  Value=JE_Brake  VectorParams1D=off  SampleTime=-1
  Constant13 : Constant  Value=JF_part_Brake  VectorParams1D=off  SampleTime=-1
  Constant14 : Constant  Value=Upd_flag  VectorParams1D=off  SampleTime=-1
  Constant15 : Constant  Value=Upd_end  VectorParams1D=off  SampleTime=-1
  Constant16 : Constant  Value=U_max  VectorParams1D=off  SampleTime=-1
  Constant2 : Constant  Value=Np  SampleTime=-1
  Constant3 : Constant  Value=JF_part  VectorParams1D=off  SampleTime=-1
  Constant4 : Constant  Value=U_min  VectorParams1D=off  SampleTime=-1
  Constant5 : Constant  Value=JF_parts  VectorParams1D=off  SampleTime=-1
  Constant6 : Constant  Value=JEs  VectorParams1D=off  SampleTime=-1
  Constant7 : Constant  Value=JE_Final  VectorParams1D=off  SampleTime=-1
  Constant8 : Constant  Value=JF_part_Final  VectorParams1D=off  SampleTime=-1
  Constant9 : Constant  Value=Ts  VectorParams1D=off  SampleTime=-1
  Demux : Demux  Outputs=3
  Digital Clock : DigitalClock  SampleTime=Ts
  Extrapolation_select : Subsystem  Commented=on
  F : Gain  Gain=F  Multiplication=Matrix(K*u) (u vector)
  F1 : Gain  Gain=F_Final  Multiplication=Matrix(K*u) (u vector)
  F_Brake : Gain  Gain=F_Brake  Multiplication=Matrix(K*u) (u vector)
  Fs : Gain  Gain=Fs  Multiplication=Matrix(K*u) (u vector)
  Mpc : MATLAB Function  TreatAsAtomicUnit=on  SystemSampleTime=Ts
  Multiport Switch : MultiPortSwitch  Inputs=4
  Multiport Switch1 : MultiPortSwitch  Inputs=4
  Multiport Switch2 : MultiPortSwitch  Inputs=4
  Mux : Mux  Inputs=3
  Mux1 : Mux  Commented=on  Inputs=3
  Switch : Switch  Commented=on  Criteria=u2 ~= 0  Threshold=Timetochange
  Unit Delay : UnitDelay  InitialCondition=[0;0]  SampleTime=Ts
  Unit Delay{1..5} (5 alike) : UnitDelay  Commented=on  InitialCondition=[0;0]  SampleTime=Ts
  U : Outport
  Ref : Outport  Port=2
  Lambda : Outport  Port=3
  wires:
  Unit Delay/1 -> Mux1/1, Mpc/19(u), Unit Delay1/1
  Rs_heading_angle/1 -> Mpc/14(Yup)
  Constant1/1 -> Mpc/6(M)
  Mpc/1(U) -> Unit Delay/1, U/1
  Constant2/1 -> Mpc/7(Np)
  Xh/1 -> F_Brake/1, F1/1, F/1, Fs/1
  Rs/1 -> Mpc/16(Rs)
  Multiport Switch1/1 -> Mpc/11(Fxh)
  Multiport Switch2/1 -> Mpc/8(JF_part)
  Constant3/1 -> Multiport Switch2/3
  Constant5/1 -> Multiport Switch2/2
  F/1 -> Multiport Switch1/3
  Fs/1 -> Multiport Switch1/2
  Multiport Switch/1 -> Mpc/2(JE)
  Constant4/1 -> Mpc/9(U_min)
  Rs_V/1 -> Mpc/13(Rs_V)
  Vup/1 -> Mpc/15(Vup)
  Rs_Y/1 -> Mpc/12(Rs_Y)
  Select/1 -> Multiport Switch1/1, Multiport Switch2/1, Multiport Switch/1
  Constant/1 -> Multiport Switch/3
  Constant6/1 -> Multiport Switch/2
  F1/1 -> Multiport Switch1/4
  Constant7/1 -> Multiport Switch/4
  Constant8/1 -> Multiport Switch2/4
  Unit Delay1/1 -> Mux1/2, Unit Delay2/1
  Constant9/1 -> Mpc/5(Ts)
  Constant10/1 -> Mpc/3(Timetochange)
  Mux/1 -> Switch/1
  Switch/1 -> Demux/1
  Mpc/4(u1) -> Unit Delay3/1
  Mpc/5(u2) -> Unit Delay4/1
  Mpc/6(u3) -> Unit Delay5/1
  Demux/1 -> Mpc/20("u1 ")
  Demux/2 -> Mpc/21("u2 ")
  Demux/3 -> Mpc/22("u3 ")
  Mux1/1 -> Switch/3
  Unit Delay2/1 -> Mux1/3
  Unit Delay3/1 -> Mux/1
  Unit Delay4/1 -> Mux/2
  Unit Delay5/1 -> Mux/3
  Extrapolation_select/1(Select) -> Switch/2
  Constant11/1 -> Mpc/4(Timetochange2)
  Constant12/1 -> Multiport Switch/5
  Constant13/1 -> Multiport Switch2/5
  F_Brake/1 -> Multiport Switch1/5
  Mpc/2(Ref) -> Ref/1
  Constant14/1 -> Mpc/1(Upd_flag)
  Constant15/1 -> Mpc/18(Upd_end)
  Digital Clock/1 -> Mpc/17(Tsim)
  Constant16/1 -> Mpc/10(U_max)
  Mpc/3(lambda) -> Lambda/1

== system Copy_of_MPC_control/all_system/Observer_state1 ==
  Clock9 : Clock
  Observer_state1 : MATLAB Function  TreatAsAtomicUnit=on  SystemSampleTime=Ts
  Timetochange : Constant  Value=Timetochange  VectorParams1D=off  SampleTime=-1
  state : Outport
  wires:
  Timetochange/1 -> Observer_state1/2(point)
  Clock9/1 -> Observer_state1/1(timing)
  Observer_state1/1(state) -> state/1

== system Copy_of_MPC_control/all_system/Observer_state2 ==
  Clock9 : Clock
  Observer_state2 : MATLAB Function  TreatAsAtomicUnit=on  SystemSampleTime=Ts
  Timetochange : Constant  Value=Earlytochange  VectorParams1D=off  SampleTime=-1
  Timetochange1 : Constant  Value=Timetochange2  VectorParams1D=off  SampleTime=-1
  state : Outport
  wires:
  Timetochange/1 -> Observer_state2/2(Earlytochange)
  Clock9/1 -> Observer_state2/1(timing)
  Observer_state2/1(state) -> state/1
  Timetochange1/1 -> Observer_state2/3(Timetochange2)

== system Copy_of_MPC_control/all_system/Observer_state3 ==
  Clock9 : Clock
  Observer_state2 : MATLAB Function  TreatAsAtomicUnit=on  SystemSampleTime=Ts
  Timetochange : Constant  Value=Earlytochange2  VectorParams1D=off  SampleTime=-1
  state : Outport
  wires:
  Timetochange/1 -> Observer_state2/2(Earlytochange2)
  Clock9/1 -> Observer_state2/1(timing)
  Observer_state2/1(state) -> state/1

== system Copy_of_MPC_control/all_system/Passenger Vehicle1 ==
  Env : Inport
  Steer : Inport  Port=2
  Cntrl : Inport  Port=3
  "Body, Suspension, Wheels" : Subsystem  Variant=on  OverrideUsingVariant=1
  Bus Creator2 : BusCreator  Inputs=4
  Engine : Subsystem  Variant=on  OverrideUsingVariant=0
  Mux : Mux  Inputs=2
  "Steering, Transmission, Driveline and Brakes" : Subsystem  Variant=on  OverrideUsingVariant=0
  Subsystem : Subsystem
  Subsystem1 : Subsystem
  Subsystem2 : Subsystem
  Subsystem3 : Subsystem
  Subsystem4 : Subsystem
  Subsystem5 : Subsystem
  Sum1 : Sum
  To Workspace1 : ToWorkspace  VariableName=yaw_sim  SampleTime=Ts
  To Workspace3 : ToWorkspace  VariableName=Beta  SampleTime=Ts
  To Workspace5 : ToWorkspace  VariableName=Velocity_tmp  SampleTime=-1
  To Workspace6 : ToWorkspace  VariableName=Velocity_y  SampleTime=-1
  beta : MATLAB Function  TreatAsAtomicUnit=on  SystemSampleTime=Tf
      settings: MinAlgLoopOccurrences=on
  VehFdbk : Outport
  Velocity : Outport  Port=2
  yaw : Outport  Port=3
  XY : Outport  Port=4
  wires:
  Bus Creator2/1 -> VehFdbk/1
  Env/1 -> Subsystem/1(Env)
  Subsystem1/1(Driveline) -> [Driveline], Bus Creator2/2  "Driveline"
  "Steering, Transmission, Driveline and Brakes"/1(WhlAng) -> Subsystem1/1(WhlAng)
  "Steering, Transmission, Driveline and Brakes"/2(AxlTrq) -> Subsystem1/2(AxlTrq)
  "Steering, Transmission, Driveline and Brakes"/3(BrkPrs) -> Subsystem1/3(BrkPrs)
  "Steering, Transmission, Driveline and Brakes"/4(EngSpd) -> Subsystem1/4(EngSpd)
  "Steering, Transmission, Driveline and Brakes"/5(PropShftSpd) -> Subsystem1/5(PropShftSpd)
  Steer/1 -> Subsystem2/2(SteerCmd)
  Cntrl/1 -> Subsystem3/1(Cntrl), Subsystem2/1(Cntrl)
  Subsystem2/1(Steer) -> "Steering, Transmission, Driveline and Brakes"/1(SteerHWCmd)
  Subsystem2/3(GearCmd) -> "Steering, Transmission, Driveline and Brakes"/3(GearCmd)
  Subsystem2/4(PrsCmd) -> "Steering, Transmission, Driveline and Brakes"/4(BrkPrsCmd)
  Subsystem2/5(omega) -> "Steering, Transmission, Driveline and Brakes"/5(omega)
  Engine/1(EngTrq) -> Subsystem5/1("EngTrq ")
  Subsystem2/2(EngTrq) -> "Steering, Transmission, Driveline and Brakes"/2(EngTrq)
  Subsystem3/1(EngTrqCmd) -> Engine/1(TrqCmd)
  Subsystem3/2(EngSpd) -> Engine/2(EngSpd)
  Subsystem4/1(Chassis) -> Bus Creator2/3  "Body"
  Subsystem4/2(Wheels) -> Bus Creator2/4, [Wheels]  "Wheels"
  Subsystem5/1(Eng) -> [EngTrq], Bus Creator2/1  "Engine"
  [Driveline] -> Subsystem/2(Driveline)
  [Wheels] -> Subsystem2/4(Wheels)
  [EngTrq] -> Subsystem2/3(EngTrqCmd)
  [Driveline] -> Subsystem3/2(Driveline)
  "Body, Suspension, Wheels"/19(XWheel) -> Subsystem4/19(XWheel)
  "Body, Suspension, Wheels"/11(p) -> Subsystem4/11(p)
  "Body, Suspension, Wheels"/12(q) -> Subsystem4/12(q)
  "Body, Suspension, Wheels"/7(Ydot) -> Subsystem4/7(Ydot)
  "Body, Suspension, Wheels"/13(r) -> Subsystem4/13(r)
  "Body, Suspension, Wheels"/16(zAxle) -> Subsystem4/16(zAxle)
  "Body, Suspension, Wheels"/8(phi) -> Subsystem4/8(phi)
  "Body, Suspension, Wheels"/3(X) -> Mux/1, Subsystem4/3(X)
  Subsystem/6(BrkPrs) -> "Body, Suspension, Wheels"/6(BrkPrs)
  "Body, Suspension, Wheels"/9(theta) -> Subsystem4/9(theta)
  "Body, Suspension, Wheels"/5(Z) -> Subsystem4/5(Z)
  Subsystem/3(mu) -> "Body, Suspension, Wheels"/3(Friction)
  "Body, Suspension, Wheels"/17(omega) -> Subsystem4/17(omega)
  Subsystem/4(WhlAng) -> "Body, Suspension, Wheels"/4(WheelAngle)
  "Body, Suspension, Wheels"/14(ay) -> Subsystem4/14(ay)
  Subsystem/1(Wind) -> "Body, Suspension, Wheels"/1(WindXYZ)
  Subsystem/2(Gnd) -> "Body, Suspension, Wheels"/2(Ground)
  "Body, Suspension, Wheels"/10(psi) -> Subsystem4/10(psi), Sum1/2
  "Body, Suspension, Wheels"/4(Y) -> Mux/2, Subsystem4/4(Y)
  Subsystem/5(AxleTrq) -> "Body, Suspension, Wheels"/5(AxleTrq)
  "Body, Suspension, Wheels"/18(ZHP) -> Subsystem4/18(ZHP)
  "Body, Suspension, Wheels"/20(YWheel) -> Subsystem4/20(YWheel)
  "Body, Suspension, Wheels"/6(Xdot) -> Subsystem4/6(Xdot)
  "Body, Suspension, Wheels"/15(kappa) -> Subsystem4/15(kappa)
  Mux/1 -> XY/1
  Sum1/1 -> yaw/1, To Workspace1/1
  beta/1(beta) -> To Workspace3/1, Sum1/1
  "Body, Suspension, Wheels"/2(ydot) -> beta/1(ydot), To Workspace6/1, Subsystem4/2(ydot)
  "Body, Suspension, Wheels"/1(xdot) -> To Workspace5/1, beta/2(xdot), Subsystem4/1(xdot)
  beta/2(Velocity) -> Velocity/1

== system Copy_of_MPC_control/all_system/Select_model1 ==
  Clock14 : Clock
  Constant2 : Constant  Value=Timetochange2
  Constant3 : Constant  Value=Timetochange
  Select_model : MATLAB Function  TreatAsAtomicUnit=on  SystemSampleTime=Ts
  Select : Outport
  wires:
  Constant3/1 -> Select_model/2(Tc1)
  Constant2/1 -> Select_model/3(Tc2)
  Clock14/1 -> Select_model/1(Time)
  Select_model/1(Select) -> Select/1

== system Copy_of_MPC_control/all_system/Simulation Interrupt 1 ==
  Y : Inport
  Abs : Abs
  Clock : Clock
  Constant : Constant
  Constant1 : Constant  Value=0
  Constant2 : Constant  Value=0
  Fcn : Fcn  Expr=u(1)
  Fcn1 : Fcn  Expr=u(1)
  From Workspace : FromWorkspace  VariableName=Rs_V_now  SampleTime=Ts
  Stop Simulation : Stop
  Sum4 : Sum  Inputs=|+-
  Switch : Switch  Threshold=1
  Switch1 : Switch  Threshold=61
  wires:
  From Workspace/1 -> Fcn1/1
  Fcn/1 -> Sum4/2
  Y/1 -> Fcn/1
  Fcn1/1 -> Sum4/1
  Switch/1 -> Switch1/3
  Sum4/1 -> Abs/1
  Clock/1 -> Switch1/2
  Constant/1 -> Switch/1
  Switch1/1 -> Stop Simulation/1
  Constant2/1 -> Switch1/1
  Abs/1 -> Switch/2
  Constant1/1 -> Switch/3

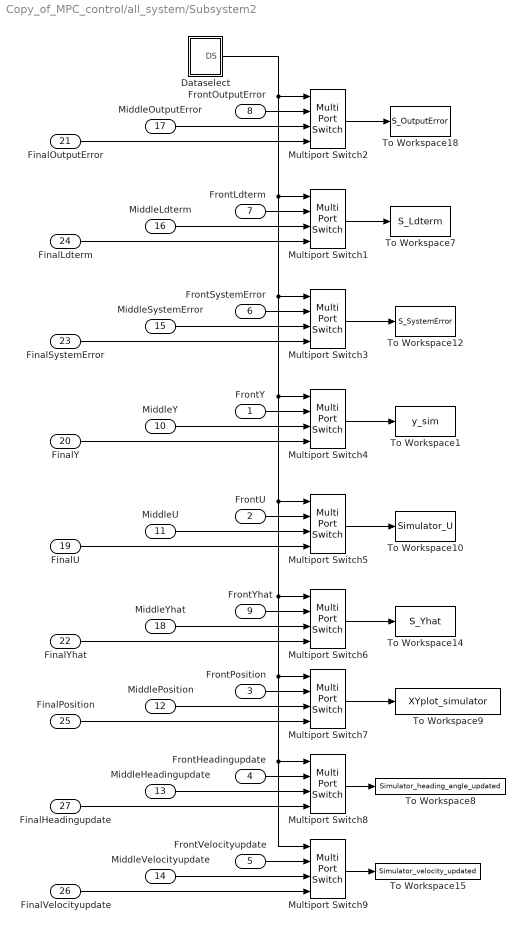
== system Copy_of_MPC_control/all_system/Subsystem2 ==
  FrontY : Inport
  FrontU : Inport  Port=2
  FrontPosition : Inport  Port=3
  FrontHeadingupdate : Inport  Port=4
  FrontVelocityupdate : Inport  Port=5
  FrontSystemError : Inport  Port=6
  FrontLdterm : Inport  Port=7
  FrontOutputError : Inport  Port=8
  FrontYhat : Inport  Port=9
  MiddleY : Inport  Port=10
  MiddleU : Inport  Port=11
  MiddlePosition : Inport  Port=12
  MiddleHeadingupdate : Inport  Port=13
  MiddleVelocityupdate : Inport  Port=14
  MiddleSystemError : Inport  Port=15
  MiddleLdterm : Inport  Port=16
  MiddleOutputError : Inport  Port=17
  MiddleYhat : Inport  Port=18
  FinalU : Inport  Port=19
  FinalY : Inport  Port=20
  FinalOutputError : Inport  Port=21
  FinalYhat : Inport  Port=22
  FinalSystemError : Inport  Port=23
  FinalLdterm : Inport  Port=24
  FinalPosition : Inport  Port=25
  FinalVelocityupdate : Inport  Port=26
  FinalHeadingupdate : Inport  Port=27
  Dataselect : Subsystem
  Multiport Switch{1..9} (9 alike) : MultiPortSwitch
  To Workspace1 : ToWorkspace  VariableName=y_sim  SampleTime=Ts
  To Workspace10 : ToWorkspace  VariableName=Simulator_U  SampleTime=Ts
  To Workspace12 : ToWorkspace  VariableName=S_SystemError  SampleTime=Ts
  To Workspace14 : ToWorkspace  VariableName=S_Yhat  SampleTime=Ts
  To Workspace15 : ToWorkspace  VariableName=Simulator_velocity_updated  SampleTime=Ts
      settings: Save2DSignal=2-D array (concatenate along first dimension)
  To Workspace18 : ToWorkspace  VariableName=S_OutputError  SampleTime=Ts
  To Workspace7 : ToWorkspace  VariableName=S_Ldterm  SampleTime=Ts
  To Workspace8 : ToWorkspace  VariableName=Simulator_heading_angle_updated  SampleTime=Ts
      settings: Save2DSignal=2-D array (concatenate along first dimension)
  To Workspace9 : ToWorkspace  VariableName=XYplot_simulator  SampleTime=Ts
  wires:
  FrontHeadingupdate/1 -> Multiport Switch8/2
  Dataselect/1(DS) -> Multiport Switch2/1, Multiport Switch7/1, Multiport Switch8/1, Multiport Switch9/1, Multiport Switch6/1, Multiport Switch5/1, Multiport Switch4/1, Multiport Switch3/1, Multiport Switch1/1
  Multiport Switch1/1 -> To Workspace7/1
  FinalSystemError/1 -> Multiport Switch3/4
  Multiport Switch4/1 -> To Workspace1/1
  Multiport Switch7/1 -> To Workspace9/1
  Multiport Switch3/1 -> To Workspace12/1
  FrontSystemError/1 -> Multiport Switch3/2
  Multiport Switch2/1 -> To Workspace18/1
  Multiport Switch5/1 -> To Workspace10/1
  FinalLdterm/1 -> Multiport Switch1/4
  FinalPosition/1 -> Multiport Switch7/4
  FrontLdterm/1 -> Multiport Switch1/2
  MiddleOutputError/1 -> Multiport Switch2/3
  FrontU/1 -> Multiport Switch5/2
  MiddleU/1 -> Multiport Switch5/3
  Multiport Switch9/1 -> To Workspace15/1
  MiddlePosition/1 -> Multiport Switch7/3
  MiddleY/1 -> Multiport Switch4/3
  Multiport Switch6/1 -> To Workspace14/1
  MiddleHeadingupdate/1 -> Multiport Switch8/3
  FrontY/1 -> Multiport Switch4/2
  FrontPosition/1 -> Multiport Switch7/2
  FinalHeadingupdate/1 -> Multiport Switch8/4
  MiddleVelocityupdate/1 -> Multiport Switch9/3
  FrontVelocityupdate/1 -> Multiport Switch9/2
  FrontOutputError/1 -> Multiport Switch2/2
  Multiport Switch8/1 -> To Workspace8/1
  MiddleSystemError/1 -> Multiport Switch3/3
  FinalOutputError/1 -> Multiport Switch2/4
  FinalU/1 -> Multiport Switch5/4
  MiddleYhat/1 -> Multiport Switch6/3
  FinalYhat/1 -> Multiport Switch6/4
  FinalY/1 -> Multiport Switch4/4
  FrontYhat/1 -> Multiport Switch6/2
  FinalVelocityupdate/1 -> Multiport Switch9/4
  MiddleLdterm/1 -> Multiport Switch1/3
